simulink library "controllable_grid_lib"  (Simulink 8.1)
settings: Solver=ode45  StartTime=0.0  StopTime=10.0  RelTol=1e-3
values from neighbouring files (symbols this model uses):
  Ts = 100E-6    (= 0.0001)    [BANSHEE_init.m]    (also in Ghost_init.m)
libraries: powerlib x5, simulink x1, powerlib_extras x1
settings Model: Creator=re25624  LastModifiedBy=pkoralew

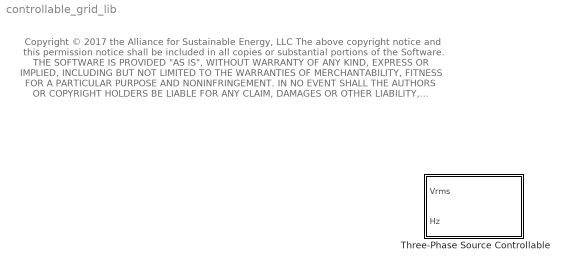
== system controllable_grid_lib ==
  note: Copyright © 2017 the Alliance for Sustainable Energy, LLC
      |
      | The above copyright notice and this permission notice shall be included in all copies or substantial portions of the Software.
      |
      | THE SOFTWARE IS PROVIDED "AS IS", WITHOUT WARRANTY OF ANY KIND, EXPRESS OR IMPLIED, INCLUDING
      | BUT NOT LIMITED TO THE WARRANTIES OF MERCHANTABILITY, FITNESS FOR A PARTICULAR PURPOSE AND
      | NONINFRINGEMENT. IN NO EVENT SHALL THE AUTHORS OR COPYRIGHT HOLDERS BE LIABLE FOR ANY CLAIM,
      |  DAMAGES OR OTHER LIABILITY, WHETHER IN AN ACTION OF CONTRACT, TORT OR OTHERWISE, ARISING FROM,
      | OUT OF OR IN CONNECTION WITH THE SOFTWARE OR THE USE OR OTHER DEALINGS IN THE SOFTWARE
  Three-Phase Source Controllable : Subsystem  mask{Ts=Ts, Rg=0.8, Lg=16.58e-3}
      mask prompts: Rg "Grid Resistance [Ohms]"; Lg "Grid Inductance [H]"

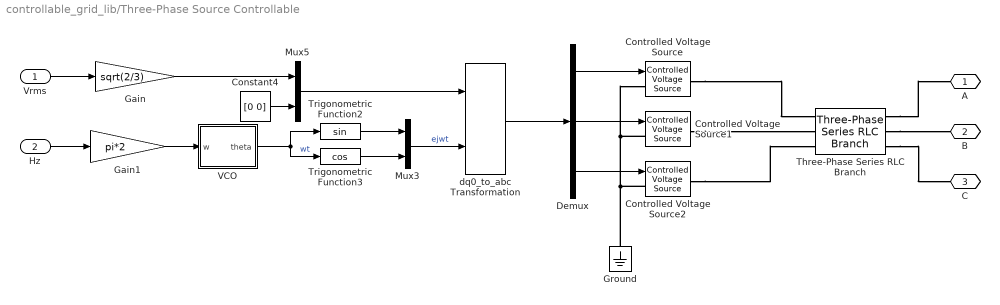
== system controllable_grid_lib/Three-Phase Source Controllable ==
  Vrms : Inport
  Hz : Inport  Port=2
  Constant4 : Constant  Value=[0 0]
  Controlled Voltage Source : powerlib/Electrical Sources/Controlled Voltage Source  Initialize=on  Source_Type=AC  Amplitude=0  Phase=0  Frequency=0  Measurements=None
  Controlled Voltage Source1 : powerlib/Electrical Sources/Controlled Voltage Source  Initialize=on  Source_Type=AC  Amplitude=0  Phase=0  Frequency=0  Measurements=None
  Controlled Voltage Source2 : powerlib/Electrical Sources/Controlled Voltage Source  Initialize=on  Source_Type=AC  Amplitude=0  Phase=0  Frequency=0  Measurements=None
  Demux : Demux  Outputs=3
  Gain : Gain  Gain=sqrt(2/3)
  Gain1 : Gain  Gain=pi*2
  Ground : powerlib/Elements/Ground  LConnTagsString=a
  Mux3 : Mux  Inputs=2
  Mux5 : Mux  Inputs=[1 2]
  Three-Phase Series RLC Branch : powerlib/Elements/Three-Phase Series RLC Branch  LConnTagsString=A|B|C  RConnTagsString=A|B|C  BranchType=RL  Resistance=Rg  Inductance=Lg  Capacitance=0  Measurements=None
  Trigonometric Function2 : Trigonometry
  Trigonometric Function3 : Trigonometry  Operator=cos
  VCO : Subsystem
  dq0_to_abc Transformation : powerlib_extras/Measurements/dq0_to_abc Transformation
  A : PMIOPort  Port=1  Side=Right
  B : PMIOPort  Port=2  Side=Right
  C : PMIOPort  Port=3  Side=Right
  wires:
  Gain1/1 -> VCO/1(w)
  Gain/1 -> Mux5/1
  Hz/1 -> Gain1/1
  VCO/1(theta) -> Trigonometric Function3/1, Trigonometric Function2/1  "wt"
  Trigonometric Function3/1 -> Mux3/2
  Mux3/1 -> dq0_to_abc Transformation/2  "ejwt"
  Demux/2 -> Controlled Voltage Source1/1
  Vrms/1 -> Gain/1
  Trigonometric Function2/1 -> Mux3/1
  dq0_to_abc Transformation/1 -> Demux/1
  Demux/1 -> Controlled Voltage Source/1
  Demux/3 -> Controlled Voltage Source2/1
  Mux5/1 -> dq0_to_abc Transformation/1
  Constant4/1 -> Mux5/2
  connections:
  Three-Phase Series RLC Branch/RConn2 -- B/RConn1
  Three-Phase Series RLC Branch/RConn3 -- C/RConn1
  Three-Phase Series RLC Branch/RConn1 -- A/RConn1
  Controlled Voltage Source2/RConn1 -- Three-Phase Series RLC Branch/LConn3
  Controlled Voltage Source1/RConn1 -- Three-Phase Series RLC Branch/LConn2
  Controlled Voltage Source2/LConn1 -- Ground/LConn1 -- Controlled Voltage Source/LConn1 -- Controlled Voltage Source1/LConn1
  Controlled Voltage Source/RConn1 -- Three-Phase Series RLC Branch/LConn1

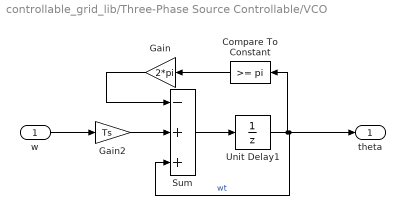
== system controllable_grid_lib/Three-Phase Source Controllable/VCO ==
  w : Inport
  Compare To Constant : simulink/Logic and Bit Operations/Compare To Constant  relop=>=  const=pi  OutDataTypeStr=uint8
  Gain : Gain  Gain=2*pi  OutDataTypeStr=double
  Gain2 : Gain  Gain=Ts  SaturateOnIntegerOverflow=on  OutDataTypeStr=Inherit: Same as input  ParamDataTypeStr=Inherit: Same as input
  Sum : Sum  Inputs=-++
  Unit Delay1 : UnitDelay  SampleTime=-1
  theta : Outport
  wires:
  Sum/1 -> Unit Delay1/1
  Gain2/1 -> Sum/2
  Unit Delay1/1 -> theta/1, Sum/3, Compare To Constant/1  "wt"
  Compare To Constant/1 -> Gain/1
  Gain/1 -> Sum/1
  w/1 -> Gain2/1
